simulink model "partSix"  (R2021b)
settings: Solver=VariableStepAuto  StartTime=0.0  StopTime=10.0  RelTol=1e-3
libraries: simulink x2
settings Model: Creator=ericp  LastModifiedBy=ericp
settings OptimizationCC: BlockReduction=off  DefaultParameterBehavior=Inlined  BufferReuse=off

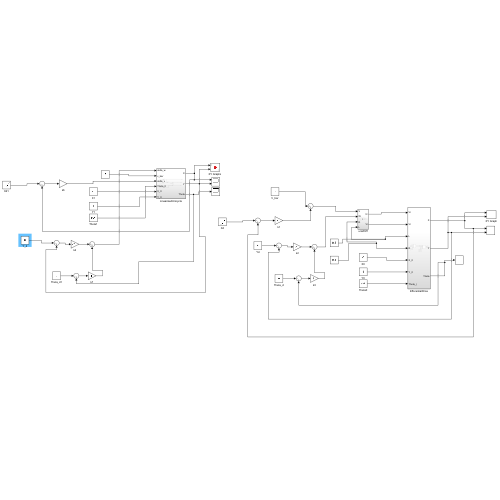
[thumbnail: Simulink's stored preview of the top-level diagram]
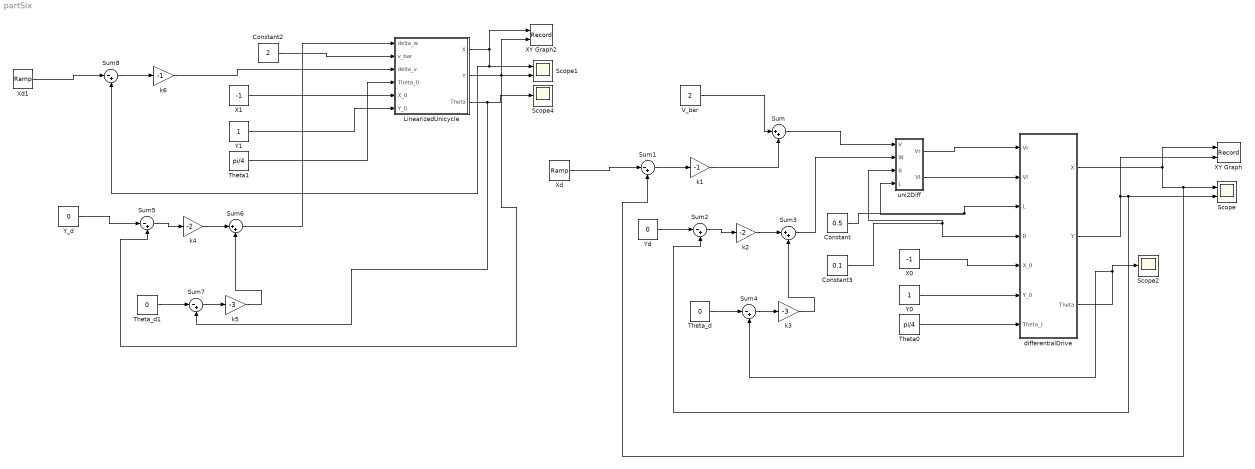
== system partSix ==
  Constant : Constant  Value=0.5
  Constant2 : Constant  Value=2
  Constant3 : Constant  Value=0.1
  LinearizedUnicycle : Subsystem
  Scope : Scope  NumInputPorts=2
  Scope1 : Scope  NumInputPorts=2
  Scope2 : Scope
  Scope4 : Scope
  Sum : Sum  Inputs=|++
  Sum{1..2,4..5,7..8} (6 alike) : Sum  Inputs=|-+
  Sum3 : Sum  Inputs=|++
  Sum6 : Sum  Inputs=|++
  Theta0 : Constant  Value=pi/4
  Theta1 : Constant  Value=pi/4
  Theta_d : Constant  Value=0
  Theta_d1 : Constant  Value=0
  V_bar : Constant  Value=2
  X0 : Constant  Value=-1
  X1 : Constant  Value=-1
  XY Graph : Record  FileSettingsInternal="{\"entries\":[{\"content\":{\"excelSettings\":{\"content\":{},\"type\":\"Streamout.ExcelSettings\"}},\"type\":\"Streamout.FileSettingStorage\",\"uuid\":\"6a5fd66f-9ecf-40f6-a285-f8fbc1d2f8f8\"}],\"packageUris\":[\"http://schema.mathworks.com/mf0/streamout_blocks/R2020a\"],\"version\":\"1.0\"}"  Layout=[1 1]  SignalsInternal="{\"entries\":[{\"content\":{\"signals\":[{\"content\":{\"blockPath\":[\"partSix/XY Graph\"],\"channel\":[],\"dimensions\":[1],\"domain\":\"partSix/XY Graph\",\"lineColor\":\"#a2142f\",\"plots\":[1],\"port\":1,\"sid\":[],\"signalID\":3380,\"signalName\":\"differentialDrive:1\"},\"type\":\"RecordBlkView.Signal\",\"uuid\":\"ab41c7fb-60eb-4fc2-975a-2cf507f883ef\"},{\"content\":{\"blockPath\":[\"partSix/XY Graph\"],\"channel\":[],\"dimensions\":[1],\"domain\":\"partSix/XY Graph\",\"lineColor\":\"#139fff\",\"plots\":[],\"port\":2,\"sid\":[],\"signalID\":3383,\"signalName\":\"differentialDrive:2\"},\"type\":\"RecordBlkView.Signal\",\"uuid\":\"2e3d908b-4035-451c-a8f8-653900188e04\"}]},\"type\":\"RecordBlkView.InputSignals\",\"uuid\":\"99ab9d17-acf3-4098-9839-47e4a43758c1\"}],\"packageUris\":[\"http://schema.mathworks.com/mf0/streamout_blocks/R2020a\"],\"version\":\"1.0\"}"  VisualizationBindings="{\"xyplotplugin\":{\"info\":[{\"series\":[],\"subplotID\":1}]}}"  CompatibilityTag=XY
  XY Graph2 : Record  FileSettingsInternal="{\"entries\":[{\"content\":{\"excelSettings\":{\"content\":{},\"type\":\"Streamout.ExcelSettings\"}},\"type\":\"Streamout.FileSettingStorage\",\"uuid\":\"875e1583-d525-4915-82c0-a9dcefed2309\"}],\"packageUris\":[\"http://schema.mathworks.com/mf0/streamout_blocks/R2020a\"],\"version\":\"1.0\"}"  Layout=[1 1]  SignalsInternal="{\"entries\":[{\"content\":{\"signals\":[{\"content\":{\"blockPath\":[\"partSix/XY Graph2\"],\"channel\":[],\"dimensions\":[1],\"domain\":\"partSix/XY Graph2\",\"lineColor\":\"#a2142f\",\"plots\":[1],\"port\":1,\"sid\":[],\"signalID\":3372,\"signalName\":\"LinearizedUnicycle:1\"},\"type\":\"RecordBlkView.Signal\",\"uuid\":\"622190c0-11ea-4261-802a-9f9d7fb7d8cb\"},{\"content\":{\"blockPath\":[\"partSix/XY Graph2\"],\"channel\":[],\"dimensions\":[1],\"domain\":\"partSix/XY Graph2\",\"lineColor\":\"#139fff\",\"plots\":[1],\"port\":2,\"sid\":[],\"signalID\":3375,\"signalName\":\"LinearizedUnicycle:2\"},\"type\":\"RecordBlkView.Signal\",\"uuid\":\"2a6695fe-a720-4ce9-954b-3b0b95894530\"}]},\"type\":\"RecordBlkView.InputSignals\",\"uuid\":\"48abd338-4bef-4cb1-9ddd-4b65753559c9\"}],\"packageUris\":[\"http://schema.mathworks.com/mf0/streamout_blocks/R2020a\"],\"version\":\"1.0\"}"  VisualizationBindings="{\"xyplotplugin\":{\"info\":[{\"series\":[{\"bindingParametersList\":[{\"parameter\":\"Y-Axis\",\"signalID\":3375,\"signalName\":\"LinearizedUnicycle:2\"},{\"parameter\":\"X-Axis\",\"signalID\":3375,\"signalName\":\"LinearizedUnicycle:2\"}],\"seriesID\":53840}],\"subplotID\":1}]}}"  CompatibilityTag=XY
  Xd : simulink/Sources/Ramp  slope=1  start=0  InitialOutput=0
  Xd1 : simulink/Sources/Ramp  slope=1  start=0  InitialOutput=0
  Y0 : Constant
  Y1 : Constant
  Y_d : Constant  Value=0
  Yd : Constant  Value=0
  differentialDrive : Subsystem
  k1 : Gain  Gain=-1
  k2 : Gain  Gain=-2
  k3 : Gain  Gain=-3
  k4 : Gain  Gain=-2
  k5 : Gain  Gain=-3
  k6 : Gain  Gain=-1
  uni2Diff : Subsystem
  wires:
  Constant3/1 -> differentialDrive/4(R), uni2Diff/3(R)
  differentialDrive/3(Theta) -> Scope2/1, Sum4/2
  Constant/1 -> uni2Diff/4(L), differentialDrive/3(L)
  differentialDrive/2(Y) -> XY Graph/2, Scope/2, Sum2/2
  differentialDrive/1(X) -> XY Graph/1, Sum1/2, Scope/1
  uni2Diff/1(Vr) -> differentialDrive/1(Vr)
  uni2Diff/2(Vl) -> differentialDrive/2(Vl)
  V_bar/1 -> Sum/1
  k1/1 -> Sum/2
  Sum1/1 -> k1/1
  Yd/1 -> Sum2/1
  Sum2/1 -> k2/1
  k2/1 -> Sum3/1
  Theta_d/1 -> Sum4/1
  Sum4/1 -> k3/1
  k3/1 -> Sum3/2
  Sum3/1 -> uni2Diff/2(W)
  Sum/1 -> uni2Diff/1(V)
  Xd/1 -> Sum1/1
  X0/1 -> differentialDrive/5(X_0)
  Y0/1 -> differentialDrive/6(Y_0)
  Theta0/1 -> differentialDrive/7(Theta_))
  Constant2/1 -> LinearizedUnicycle/2(v_bar)
  Theta1/1 -> LinearizedUnicycle/4(Theta_0)
  Y1/1 -> LinearizedUnicycle/6(Y_0)
  X1/1 -> LinearizedUnicycle/5(X_0)
  LinearizedUnicycle/3(Theta) -> Sum7/2, Scope4/1
  k5/1 -> Sum6/2
  Sum6/1 -> LinearizedUnicycle/1(delta_w)
  LinearizedUnicycle/2(Y) -> Sum5/2, XY Graph2/2, Scope1/2
  Sum5/1 -> k4/1
  Theta_d1/1 -> Sum7/1
  Sum7/1 -> k5/1
  k4/1 -> Sum6/1
  Y_d/1 -> Sum5/1
  Sum8/1 -> k6/1
  k6/1 -> LinearizedUnicycle/3(delta_v)
  LinearizedUnicycle/1(X) -> XY Graph2/1, Scope1/1, Sum8/2
  Xd1/1 -> Sum8/1

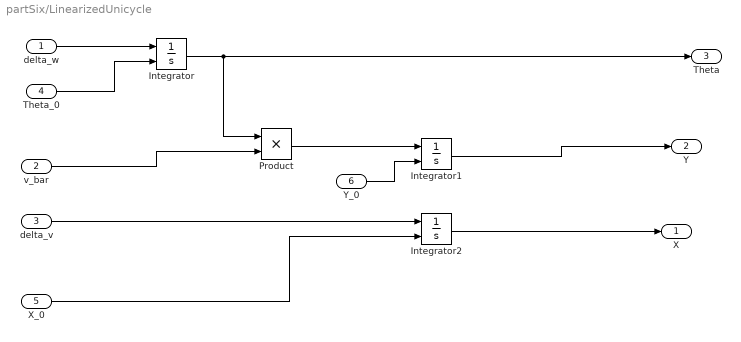
== system partSix/LinearizedUnicycle ==
  delta_w : Inport
  v_bar : Inport  Port=2
  delta_v : Inport  Port=3
  Theta_0 : Inport  Port=4
  X_0 : Inport  Port=5
  Y_0 : Inport  Port=6
  Integrator : Integrator  InitialConditionSource=external
  Integrator1 : Integrator  InitialConditionSource=external
  Integrator2 : Integrator  InitialConditionSource=external
  Product : Product
  X : Outport
  Y : Outport  Port=2
  Theta : Outport  Port=3
  wires:
  Integrator/1 -> Theta/1, Product/1
  Theta_0/1 -> Integrator/2
  v_bar/1 -> Product/2
  Product/1 -> Integrator1/1
  delta_w/1 -> Integrator/1
  X_0/1 -> Integrator2/2
  Integrator1/1 -> Y/1
  Y_0/1 -> Integrator1/2
  delta_v/1 -> Integrator2/1
  Integrator2/1 -> X/1

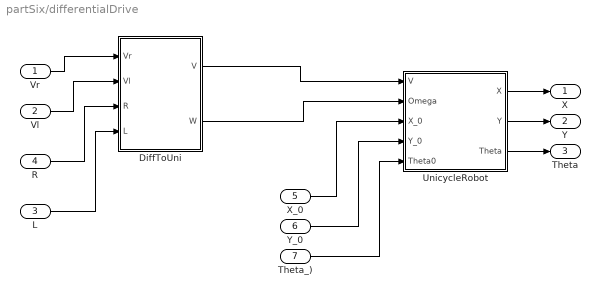
== system partSix/differentialDrive ==
  Vr : Inport
  Vl : Inport  Port=2
  L : Inport  Port=3
  R : Inport  Port=4
  X_0 : Inport  Port=5
  Y_0 : Inport  Port=6
  Theta_) : Inport  Port=7
  DiffToUni : Subsystem
  UnicycleRobot : Subsystem
  X : Outport
  Y : Outport  Port=2
  Theta : Outport  Port=3
  wires:
  Y_0/1 -> UnicycleRobot/4(Y_0)
  UnicycleRobot/3(Theta) -> Theta/1
  UnicycleRobot/1(X) -> X/1
  UnicycleRobot/2(Y) -> Y/1
  DiffToUni/1(V) -> UnicycleRobot/1(V)
  Theta_)/1 -> UnicycleRobot/5(Theta0)
  Vr/1 -> DiffToUni/1(Vr)
  DiffToUni/2(W) -> UnicycleRobot/2(Omega)
  R/1 -> DiffToUni/3(R)
  Vl/1 -> DiffToUni/2(Vl)
  L/1 -> DiffToUni/4(L)
  X_0/1 -> UnicycleRobot/3(X_0)

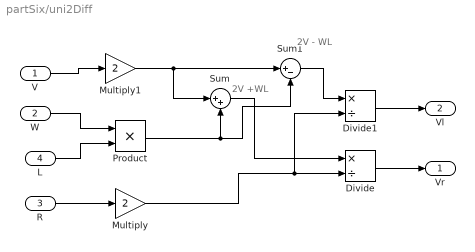
== system partSix/uni2Diff ==
  note: 2V +WL
  note: 2V - WL
  V : Inport
  W : Inport  Port=2
  R : Inport  Port=3
  L : Inport  Port=4
  Divide : Product  Inputs=*/
  Divide1 : Product  Inputs=*/
  Multiply : Gain  Gain=2
  Multiply1 : Gain  Gain=2
  Product : Product
  Sum : Sum  Inputs=|++
  Sum1 : Sum  Inputs=|+-
  Vr : Outport
  Vl : Outport  Port=2
  wires:
  V/1 -> Multiply1/1
  Divide/1 -> Vr/1
  Sum1/1 -> Divide1/1
  Multiply/1 -> Divide1/2, Divide/2
  Divide1/1 -> Vl/1
  L/1 -> Product/2
  R/1 -> Multiply/1
  Multiply1/1 -> Sum1/1, Sum/1
  Sum/1 -> Divide/1
  Product/1 -> Sum1/2, Sum/2
  W/1 -> Product/1

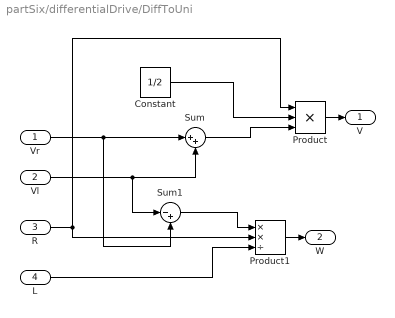
== system partSix/differentialDrive/DiffToUni ==
  Vr : Inport
  Vl : Inport  Port=2
  R : Inport  Port=3
  L : Inport  Port=4
  Constant : Constant  Value=1/2
  Product : Product  Inputs=3
  Product1 : Product  Inputs=**/  InputSameDT=on
  Sum : Sum  Inputs=|++
  Sum1 : Sum  Inputs=|-+
  V : Outport
  W : Outport  Port=2
  wires:
  Vl/1 -> Sum1/1, Sum/2
  L/1 -> Product1/3
  Sum/1 -> Product/3
  Vr/1 -> Sum1/2, Sum/1
  R/1 -> Product1/2, Product/1
  Constant/1 -> Product/2
  Sum1/1 -> Product1/1
  Product/1 -> V/1
  Product1/1 -> W/1

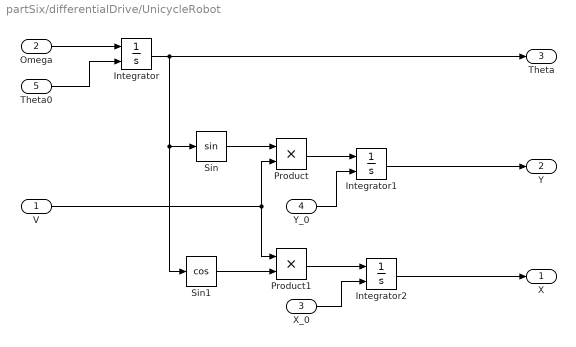
== system partSix/differentialDrive/UnicycleRobot ==
  V : Inport
  Omega : Inport  Port=2
  X_0 : Inport  Port=3
  Y_0 : Inport  Port=4
  Theta0 : Inport  Port=5
  Integrator : Integrator  InitialConditionSource=external
  Integrator1 : Integrator  InitialConditionSource=external
  Integrator2 : Integrator  InitialConditionSource=external
  Product : Product
  Product1 : Product
  Sin : Trigonometry
  Sin1 : Trigonometry  Operator=cos
  X : Outport
  Y : Outport  Port=2
  Theta : Outport  Port=3
  wires:
  Sin1/1 -> Product1/2
  V/1 -> Product1/1, Product/2
  Integrator/1 -> Theta/1, Sin1/1, Sin/1
  Integrator2/1 -> X/1
  Sin/1 -> Product/1
  Theta0/1 -> Integrator/2
  Y_0/1 -> Integrator1/2
  Omega/1 -> Integrator/1
  X_0/1 -> Integrator2/2
  Integrator1/1 -> Y/1
  Product1/1 -> Integrator2/1
  Product/1 -> Integrator1/1
